simulink model "mrefrobotarm_modified_previous_y_previous_u_previous_ref"  (R2018b)
settings: Solver=FixedStepAuto  StartTime=0.0  StopTime=10  RelTol=1e-3  AbsTol=1e-6
undefined symbols (not defined in the file or in its folder): options, sfunxy2
libraries: neural x949, simulink x1
(part 10 of 31)

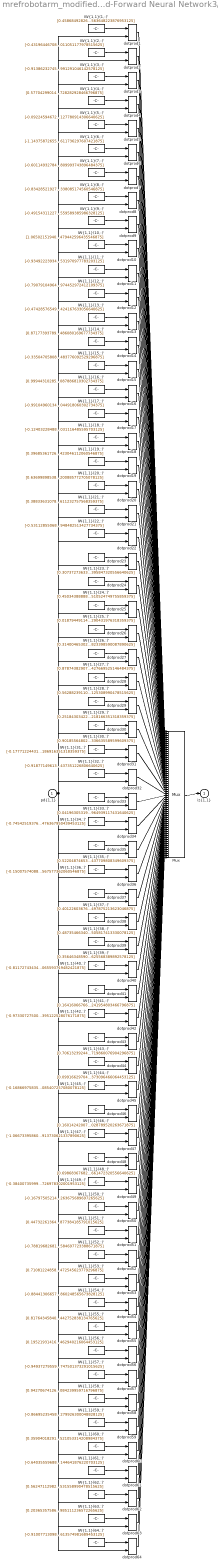
== system mrefrobotarm_modified_previous_y_previous_u_previous_ref/Feed-Forward Neural Network3/Layer 1/IW{1,1} ==
  "pd{1,1}" : Inport  PortDimensions=10
      mask Display: e = 0.06;c1 = [120 230 180]/255;c2 = ([120 230 180]+0)/(256+128);c3 = ([120 230 180]+128)/(256+128);patch([0 1 1 0],[0 0 1 1],c1);patch([0 1 1 1-e 1-e 0+e],[0 0 1 1-e 0+e 0+e],c2);patch([0 0 1 1-e 0+e 0+e],[0 1 1 1-e 1-e 0+e],c3);plot([0 1 1 0 0],[0 0 1 1 0]);
  "IW{1,1}(1,:)'" : Constant  Value=[0.45868492826623252778261985440622083842754364013671875;0.92289285731776471433107644770643673837184906005859375;-0.9045151079076070299578304911847226321697235107421875;0.6809770305948614765867432652157731354236602783203125;0.087608306906038213579535067765391431748867034912109375;-0.66859815839908964818505410221405327320098876953125;0.59153382468235282676261022061225958168506622314453125;0.66963699792932296350755905223195441067218780517578125;-0.464262938377100364828464762467774562537670135498046875;0.56319562975735781851227557126549072563648223876953125]
      mask Display: e = 0.06;c1 = [120 150 230]/255;c2 = ([120 150 230]+0)/383;c3 = ([120 150 230]+128)/383;patch([0 1 1 0],[0 0 1 1],c1);patch([0 1 1 1-e 1-e 0+e],[0 0 1 1-e 0+e 0+e],c2);patch([0 0 1 1-e 0+e 0+e],[0 1 1 1-e 1-e 0+e],c3);plot([0 1 1 0 0],[0 0 1 1 0]);disp('Weights');
  "IW{1,1}(10,:)'" : Constant  Value=[1.0650215194068157753548575783497653901576995849609375;0.923145532654704226160902180708944797515869140625;-0.28571602112830019049027896471670828759670257568359375;0.2206176877894590881989955732933594845235347747802734375;0.391759031266789181646714723683544434607028961181640625;0.4150000499566035561116450480767525732517242431640625;0.860171860662010789866371851530857384204864501953125;0.0858881248601063573833158670822740532457828521728515625;0.5686673804248325581056633382104337215423583984375;-0.8955203949568850685380994036677293479442596435546875]
      mask Display: e = 0.06;c1 = [120 150 230]/255;c2 = ([120 150 230]+0)/383;c3 = ([120 150 230]+128)/383;patch([0 1 1 0],[0 0 1 1],c1);patch([0 1 1 1-e 1-e 0+e],[0 0 1 1-e 0+e 0+e],c2);patch([0 0 1 1-e 0+e 0+e],[0 1 1 1-e 1-e 0+e],c3);plot([0 1 1 0 0],[0 0 1 1 0]);disp('Weights');
  "IW{1,1}(11,:)'" : Constant  Value=[-0.93492223934107243632496420104871504008769989013671875;0.356879505478416347852288481590221635997295379638671875;-0.042209624670428151638201796913563157431781291961669921875;0.6022490918690073247176997028873302042484283447265625;-1.3686982846566972948920692942920140922069549560546875;0.40979658750527558908061109832488000392913818359375;0.1714981863599602529557586194641771726310253143310546875;-0.75640045003631828368639844484278000891208648681640625;-0.12006348380912713891266463406282127834856510162353515625;0.632123796732191323144434136338531970977783203125]
      mask Display: e = 0.06;c1 = [120 150 230]/255;c2 = ([120 150 230]+0)/383;c3 = ([120 150 230]+128)/383;patch([0 1 1 0],[0 0 1 1],c1);patch([0 1 1 1-e 1-e 0+e],[0 0 1 1-e 0+e 0+e],c2);patch([0 0 1 1-e 0+e 0+e],[0 1 1 1-e 1-e 0+e],c3);plot([0 1 1 0 0],[0 0 1 1 0]);disp('Weights');
  "IW{1,1}(12,:)'" : Constant  Value=[-0.790791049648713606501360118272714316844940185546875;1.636635942456649228660126027534715831279754638671875;0.1645966634930366712108451565654831938445568084716796875;0.423800984374966327461464743464603088796138763427734375;-0.480947159258651557589558933614171110093593597412109375;-0.336459083953336790528965138946659862995147705078125;-0.29103815338116156841152815104578621685504913330078125;0.36537606798097732596630748957977630198001861572265625;0.5351649818216219767208485791343264281749725341796875;-0.360421095733105933955897626219666562974452972412109375]
      mask Display: e = 0.06;c1 = [120 150 230]/255;c2 = ([120 150 230]+0)/383;c3 = ([120 150 230]+128)/383;patch([0 1 1 0],[0 0 1 1],c1);patch([0 1 1 1-e 1-e 0+e],[0 0 1 1-e 0+e 0+e],c2);patch([0 0 1 1-e 0+e 0+e],[0 1 1 1-e 1-e 0+e],c3);plot([0 1 1 0 0],[0 0 1 1 0]);disp('Weights');
  "IW{1,1}(13,:)'" : Constant  Value=[-0.47428576549192869027393726355512626469135284423828125;0.481480766900708678779352567289606668055057525634765625;0.73462601397020887983302372958860360085964202880859375;-0.759579012370747985727348350337706506252288818359375;-2.289916762842977959735435433685779571533203125;-0.1033609967207107793729647937652771361172199249267578125;-1.0397695114935359139707315989653579890727996826171875;-0.11461751153739645203710750820391695015132427215576171875;0.607068239082933391870255945832468569278717041015625;0.627700190232618471242176383384503424167633056640625]
      mask Display: e = 0.06;c1 = [120 150 230]/255;c2 = ([120 150 230]+0)/383;c3 = ([120 150 230]+128)/383;patch([0 1 1 0],[0 0 1 1],c1);patch([0 1 1 1-e 1-e 0+e],[0 0 1 1-e 0+e 0+e],c2);patch([0 0 1 1-e 0+e 0+e],[0 1 1 1-e 1-e 0+e],c3);plot([0 1 1 0 0],[0 0 1 1 0]);disp('Weights');
  "IW{1,1}(14,:)'" : Constant  Value=[0.87177393789064960838430806688847951591014862060546875;-0.4062935623759871273108501554816029965877532958984375;-0.184561604501509435305450779196689836680889129638671875;-0.30955013114295903964290346266352571547031402587890625;-1.07748704376167214746828904026187956333160400390625;0.5280876054022181076419428791268728673458099365234375;-0.9211683717671104165702899990719743072986602783203125;0.4257168604823367008549439560738392174243927001953125;-0.9567072022642946205195357833872549235820770263671875;0.72989237124469974471452360376133583486080169677734375]
      mask Display: e = 0.06;c1 = [120 150 230]/255;c2 = ([120 150 230]+0)/383;c3 = ([120 150 230]+128)/383;patch([0 1 1 0],[0 0 1 1],c1);patch([0 1 1 1-e 1-e 0+e],[0 0 1 1-e 0+e 0+e],c2);patch([0 0 1 1-e 0+e 0+e],[0 1 1 1-e 1-e 0+e],c3);plot([0 1 1 0 0],[0 0 1 1 0]);disp('Weights');
  "IW{1,1}(15,:)'" : Constant  Value=[-0.335047058088355165228477972050313837826251983642578125;0.20537436519986662641912289473111741244792938232421875;-0.370389460774058376646422630074084736406803131103515625;-1.0764725130322230217672085927915759384632110595703125;0.9400904265613887478281185394735075533390045166015625;-0.90491999311588988685883805374032817780971527099609375;0.270630872633476904365323889578576199710369110107421875;0.7130288673092282092369487145333550870418548583984375;0.635657126622342527610953766270540654659271240234375;0.049580374452241053606638132578154909424483776092529296875]
      mask Display: e = 0.06;c1 = [120 150 230]/255;c2 = ([120 150 230]+0)/383;c3 = ([120 150 230]+128)/383;patch([0 1 1 0],[0 0 1 1],c1);patch([0 1 1 1-e 1-e 0+e],[0 0 1 1-e 0+e 0+e],c2);patch([0 0 1 1-e 0+e 0+e],[0 1 1 1-e 1-e 0+e],c3);plot([0 1 1 0 0],[0 0 1 1 0]);disp('Weights');
  "IW{1,1}(16,:)'" : Constant  Value=[0.9994431028540848860330925162998028099536895751953125;-0.07201816354893468552500479518130305223166942596435546875;0.9869266919961894313217953822459094226360321044921875;-0.037193845598922033179878354758329805918037891387939453125;0.0896492565684388897917500571566051803529262542724609375;0.030134033081079487914610837151485611684620380401611328125;0.57507766525746728536461205294472165405750274658203125;0.95965429457013395886377793431165628135204315185546875;-0.65200310057389998519283835776150226593017578125;0.7715891597542761104477904154919087886810302734375]
      mask Display: e = 0.06;c1 = [120 150 230]/255;c2 = ([120 150 230]+0)/383;c3 = ([120 150 230]+128)/383;patch([0 1 1 0],[0 0 1 1],c1);patch([0 1 1 1-e 1-e 0+e],[0 0 1 1-e 0+e 0+e],c2);patch([0 0 1 1-e 0+e 0+e],[0 1 1 1-e 1-e 0+e],c3);plot([0 1 1 0 0],[0 0 1 1 0]);disp('Weights');
  "IW{1,1}(17,:)'" : Constant  Value=[-0.991049601348017450419547458295710384845733642578125;0.1767823626110802404109989538483205251395702362060546875;-0.77042637580729300683657356785261072218418121337890625;1.0369587591067332965621972107328474521636962890625;-0.8204067837491482162448619419592432677745819091796875;-0.8007430151625019032479713132488541305065155029296875;0.09562009879907318321556886075995862483978271484375;-0.55794220575710007370417997663025744259357452392578125;0.663058379158372179773550669779069721698760986328125;0.12039199732993309532869119493625476025044918060302734375]
      mask Display: e = 0.06;c1 = [120 150 230]/255;c2 = ([120 150 230]+0)/383;c3 = ([120 150 230]+128)/383;patch([0 1 1 0],[0 0 1 1],c1);patch([0 1 1 1-e 1-e 0+e],[0 0 1 1-e 0+e 0+e],c2);patch([0 0 1 1-e 0+e 0+e],[0 1 1 1-e 1-e 0+e],c3);plot([0 1 1 0 0],[0 0 1 1 0]);disp('Weights');
  "IW{1,1}(18,:)'" : Constant  Value=[-0.12403228488311750232764296697496320120990276336669921875;-0.856750459537330311121650083805434405803680419921875;0.192918443102331804706039974917075596749782562255859375;1.03664335999274204169751101289875805377960205078125;-0.246904966516503676654537002832512371242046356201171875;-1.04666463077165872164187021553516387939453125;-0.033336987951685347064678666129111661575734615325927734375;0.855943230966101253898159484378993511199951171875;0.249998464760956162766802890473627485334873199462890625;0.71561037633987834016835449801874347031116485595703125]
      mask Display: e = 0.06;c1 = [120 150 230]/255;c2 = ([120 150 230]+0)/383;c3 = ([120 150 230]+128)/383;patch([0 1 1 0],[0 0 1 1],c1);patch([0 1 1 1-e 1-e 0+e],[0 0 1 1-e 0+e 0+e],c2);patch([0 0 1 1-e 0+e 0+e],[0 1 1 1-e 1-e 0+e],c3);plot([0 1 1 0 0],[0 0 1 1 0]);disp('Weights');
  "IW{1,1}(19,:)'" : Constant  Value=[0.39685361726252110781132387273828499019145965576171875;-0.7385100253306242645834345239563845098018646240234375;-0.032023900811615581274427455582554102875292301177978515625;-1.0360471954462855403988896796363405883312225341796875;0.024414108875345917615273805267861462198197841644287109375;-0.54557027817496128729857218786492012441158294677734375;-0.825321885041145009154206491075456142425537109375;-0.4206523039094769433887677223538048565387725830078125;-0.9226889362967900520828834487474523484706878662109375;0.5855123554608023805911898307385854423046112060546875]
      mask Display: e = 0.06;c1 = [120 150 230]/255;c2 = ([120 150 230]+0)/383;c3 = ([120 150 230]+128)/383;patch([0 1 1 0],[0 0 1 1],c1);patch([0 1 1 1-e 1-e 0+e],[0 0 1 1-e 0+e 0+e],c2);patch([0 0 1 1-e 0+e 0+e],[0 1 1 1-e 1-e 0+e],c3);plot([0 1 1 0 0],[0 0 1 1 0]);disp('Weights');
  "IW{1,1}(2,:)'" : Constant  Value=[-0.4319644670862052837634337265626527369022369384765625;1.131663563801270644404439735808409750461578369140625;-0.3687061577706416404254241570015437901020050048828125;-0.366144655751171221869100236290250904858112335205078125;-1.1602768057870693763078406846034340560436248779296875;0.1935191644854985237866884517643484286963939666748046875;-1.1688198788845378661704899059259332716464996337890625;0.59642228088652526896140670942259021103382110595703125;-0.213316011820075479565872456078068353235721588134765625;-0.60843334155029238363709964687586762011051177978515625]
      mask Display: e = 0.06;c1 = [120 150 230]/255;c2 = ([120 150 230]+0)/383;c3 = ([120 150 230]+128)/383;patch([0 1 1 0],[0 0 1 1],c1);patch([0 1 1 1-e 1-e 0+e],[0 0 1 1-e 0+e 0+e],c2);patch([0 0 1 1-e 0+e 0+e],[0 1 1 1-e 1-e 0+e],c3);plot([0 1 1 0 0],[0 0 1 1 0]);disp('Weights');
  "IW{1,1}(20,:)'" : Constant  Value=[0.63699898538872490316720131886540912091732025146484375;1.22411360040730965437205668422393500804901123046875;-0.2390034119129008927107093995800823904573917388916015625;-0.4946309213569535234711338489432819187641143798828125;-0.310348111937733095455627108094631694257259368896484375;0.64481659009713354624437897655298002064228057861328125;-0.406894473883987861650979311889386735856533050537109375;-0.75915863551750917270766194633324630558490753173828125;-0.9316675248445800416874362781527452170848846435546875;0.4791981902970114948203672611271031200885772705078125]
      mask Display: e = 0.06;c1 = [120 150 230]/255;c2 = ([120 150 230]+0)/383;c3 = ([120 150 230]+128)/383;patch([0 1 1 0],[0 0 1 1],c1);patch([0 1 1 1-e 1-e 0+e],[0 0 1 1-e 0+e 0+e],c2);patch([0 0 1 1-e 0+e 0+e],[0 1 1 1-e 1-e 0+e],c3);plot([0 1 1 0 0],[0 0 1 1 0]);disp('Weights');
  "IW{1,1}(21,:)'" : Constant  Value=[0.38833631078315045126458926461054943501949310302734375;-0.477922123057430703330084043045644648373126983642578125;-0.480202975146608534995351647012284956872463226318359375;-0.55323452941971229535056409076787531375885009765625;0.9656831493714037595310628603328950703144073486328125;-0.77207012724652568369521077329409308731555938720703125;0.819346846772037284978296156623400747776031494140625;1.237663352466707333832118820282630622386932373046875;-0.33134863320223384430818214241298846900463104248046875;-0.3405186420123695878459102459601126611232757568359375]
      mask Display: e = 0.06;c1 = [120 150 230]/255;c2 = ([120 150 230]+0)/383;c3 = ([120 150 230]+128)/383;patch([0 1 1 0],[0 0 1 1],c1);patch([0 1 1 1-e 1-e 0+e],[0 0 1 1-e 0+e 0+e],c2);patch([0 0 1 1-e 0+e 0+e],[0 1 1 1-e 1-e 0+e],c3);plot([0 1 1 0 0],[0 0 1 1 0]);disp('Weights');
  "IW{1,1}(22,:)'" : Constant  Value=[-0.53112855068060838004129209366510622203350067138671875;0.41770532386455538897962469491176307201385498046875;0.877645280928558424449192898464389145374298095703125;0.71215987560110016740821947678341530263423919677734375;-0.762781721122099298781904508359730243682861328125;0.5052308643133749388454134532366879284381866455078125;0.70107445065553763985377599965431727468967437744140625;0.9375496189941594504801969378604553639888763427734375;0.1867677108731029267385537195877986960113048553466796875;0.65377202488005303759877051561488769948482513427734375]
      mask Display: e = 0.06;c1 = [120 150 230]/255;c2 = ([120 150 230]+0)/383;c3 = ([120 150 230]+128)/383;patch([0 1 1 0],[0 0 1 1],c1);patch([0 1 1 1-e 1-e 0+e],[0 0 1 1-e 0+e 0+e],c2);patch([0 0 1 1-e 0+e 0+e],[0 1 1 1-e 1-e 0+e],c3);plot([0 1 1 0 0],[0 0 1 1 0]);disp('Weights');
  "IW{1,1}(23,:)'" : Constant  Value=[0.307372736331202711657084591934108175337314605712890625;-0.05892926126433717382013810492935590445995330810546875;-0.8454741438367745498538852189085446298122406005859375;-0.90214871964219345290558749184128828346729278564453125;0.52882827674761923031354626800748519599437713623046875;-0.91735938960778806716689359745942056179046630859375;0.439037397626755587776159472923609428107738494873046875;-0.8401705313617597870035069718142040073871612548828125;-0.68098266724226419466248216849635355174541473388671875;-0.6560593294393444185885755359777249395847320556640625]
      mask Display: e = 0.06;c1 = [120 150 230]/255;c2 = ([120 150 230]+0)/383;c3 = ([120 150 230]+128)/383;patch([0 1 1 0],[0 0 1 1],c1);patch([0 1 1 1-e 1-e 0+e],[0 0 1 1-e 0+e 0+e],c2);patch([0 0 1 1-e 0+e 0+e],[0 1 1 1-e 1-e 0+e],c3);plot([0 1 1 0 0],[0 0 1 1 0]);disp('Weights');
  "IW{1,1}(24,:)'" : Constant  Value=[0.4503438888826376551577368445578031241893768310546875;0.7786736499867739080826822828385047614574432373046875;-0.1252306288409761325652880259440280497074127197265625;-0.377179788931731818646397869088104926049709320068359375;0.56682512736796419883233966174884699285030364990234375;0.7596722035946166240449883844121359288692474365234375;-1.1299355991591040204724549766979180276393890380859375;-0.30400712082542213909874817545642144978046417236328125;1.0664004939714619712987087041256017982959747314453125;-0.20735732554729435772600254495046101510524749755859375]
      mask Display: e = 0.06;c1 = [120 150 230]/255;c2 = ([120 150 230]+0)/383;c3 = ([120 150 230]+128)/383;patch([0 1 1 0],[0 0 1 1],c1);patch([0 1 1 1-e 1-e 0+e],[0 0 1 1-e 0+e 0+e],c2);patch([0 0 1 1-e 0+e 0+e],[0 1 1 1-e 1-e 0+e],c3);plot([0 1 1 0 0],[0 0 1 1 0]);disp('Weights');
  "IW{1,1}(25,:)'" : Constant  Value=[0.0187944911497716395099022435033475630916655063629150390625;-0.29171160022622633078981380094774067401885986328125;-0.6290327137339668528426273041986860334873199462890625;-0.60111063940849718267855905651231296360492706298828125;-0.84503479054379526669293909435509704053401947021484375;1.00065376837120112440970842726528644561767578125;-1.0220616759307910026421950533404015004634857177734375;0.23813155884114645122195952353649772703647613525390625;0.58258232582170721425285364603041671216487884521484375;-0.2077397536722867810166093249790719710290431976318359375]
      mask Display: e = 0.06;c1 = [120 150 230]/255;c2 = ([120 150 230]+0)/383;c3 = ([120 150 230]+128)/383;patch([0 1 1 0],[0 0 1 1],c1);patch([0 1 1 1-e 1-e 0+e],[0 0 1 1-e 0+e 0+e],c2);patch([0 0 1 1-e 0+e 0+e],[0 1 1 1-e 1-e 0+e],c3);plot([0 1 1 0 0],[0 0 1 1 0]);disp('Weights');
  "IW{1,1}(26,:)'" : Constant  Value=[0.314004653024913926717687218115315772593021392822265625;0.28496225052615298256597498038900084793567657470703125;-0.020555819018938083220238155490733333863317966461181640625;-0.768406212368593966033358810818754136562347412109375;-0.702615478109754665325681344256736338138580322265625;-1.189394172537658445065744672319851815700531005859375;-0.90344082742903542015966422695782966911792755126953125;-0.282389771335746553315715345888747833669185638427734375;0.06348411509587427448142449293300160206854343414306640625;0.3946538105354913117395199151360429823398590087890625]
      mask Display: e = 0.06;c1 = [120 150 230]/255;c2 = ([120 150 230]+0)/383;c3 = ([120 150 230]+128)/383;patch([0 1 1 0],[0 0 1 1],c1);patch([0 1 1 1-e 1-e 0+e],[0 0 1 1-e 0+e 0+e],c2);patch([0 0 1 1-e 0+e 0+e],[0 1 1 1-e 1-e 0+e],c3);plot([0 1 1 0 0],[0 0 1 1 0]);disp('Weights');
  "IW{1,1}(27,:)'" : Constant  Value=[0.87874382907473036485868078671046532690525054931640625;0.60810217822310008717323626115103252232074737548828125;-0.292770568818674081779107609690981917083263397216796875;-1.0529162479607714342222379855229519307613372802734375;-0.65486630135451984191519159139716066420078277587890625;-0.797220628919749874086164709297008812427520751953125;0.1839437904078597696422292528950492851436138153076171875;-0.1829250381180290430105372934121987782418727874755859375;-0.333508322957326963642543660171213559806346893310546875;0.73330763357021933046553385793231427669525146484375]
      mask Display: e = 0.06;c1 = [120 150 230]/255;c2 = ([120 150 230]+0)/383;c3 = ([120 150 230]+128)/383;patch([0 1 1 0],[0 0 1 1],c1);patch([0 1 1 1-e 1-e 0+e],[0 0 1 1-e 0+e 0+e],c2);patch([0 0 1 1-e 0+e 0+e],[0 1 1 1-e 1-e 0+e],c3);plot([0 1 1 0 0],[0 0 1 1 0]);disp('Weights');
  "IW{1,1}(28,:)'" : Constant  Value=[0.56288239110132021192356432948145084083080291748046875;-0.9167817868636156664052805354003794491291046142578125;-0.37108127426537418358520881156437098979949951171875;-0.94968441008708370798530040701734833419322967529296875;-0.828961314456096776126514669158495962619781494140625;-0.34260164506463797184920849758782424032688140869140625;0.56198258845486204204888736057910136878490447998046875;0.463369775931001648405782589179580099880695343017578125;0.89346008209063698668472852659760974347591400146484375;-0.37152484249957906659034279073239304125308990478515625]
      mask Display: e = 0.06;c1 = [120 150 230]/255;c2 = ([120 150 230]+0)/383;c3 = ([120 150 230]+128)/383;patch([0 1 1 0],[0 0 1 1],c1);patch([0 1 1 1-e 1-e 0+e],[0 0 1 1-e 0+e 0+e],c2);patch([0 0 1 1-e 0+e 0+e],[0 1 1 1-e 1-e 0+e],c3);plot([0 1 1 0 0],[0 0 1 1 0]);disp('Weights');
  "IW{1,1}(29,:)'" : Constant  Value=[0.251843034229094986375940834477660246193408966064453125;-0.307514231193741272019082089173025451600551605224609375;1.017125500204711929796985714347101747989654541015625;0.460524441656800342936861625275923870503902435302734375;0.79131721944803856683137155414442531764507293701171875;0.57246841923376201588524736507679335772991180419921875;0.7128468337145701383406048989854753017425537109375;-0.63645636262505400626565688071423210203647613525390625;-0.74370154532832533078590131481178104877471923828125;0.32549381312921976672214441350661218166351318359375]
      mask Display: e = 0.06;c1 = [120 150 230]/255;c2 = ([120 150 230]+0)/383;c3 = ([120 150 230]+128)/383;patch([0 1 1 0],[0 0 1 1],c1);patch([0 1 1 1-e 1-e 0+e],[0 0 1 1-e 0+e 0+e],c2);patch([0 0 1 1-e 0+e 0+e],[0 1 1 1-e 1-e 0+e],c3);plot([0 1 1 0 0],[0 0 1 1 0]);disp('Weights');
  "IW{1,1}(3,:)'" : Constant  Value=[-0.91386232745777451480506670122849754989147186279296875;-0.45074517661076374253070753184147179126739501953125;0.7779681185418085842542268437682650983333587646484375;0.301880156597266358087239268570556305348873138427734375;-0.36510036078684515725711889899685047566890716552734375;0.435149932138041872775602314504794776439666748046875;0.744516076638678470089871552772819995880126953125;0.79936263013440156388611512738862074911594390869140625;-0.9761044371817184650552690072800032794475555419921875;0.09260100631979346907929340204645995981991291046142578125]
      mask Display: e = 0.06;c1 = [120 150 230]/255;c2 = ([120 150 230]+0)/383;c3 = ([120 150 230]+128)/383;patch([0 1 1 0],[0 0 1 1],c1);patch([0 1 1 1-e 1-e 0+e],[0 0 1 1-e 0+e 0+e],c2);patch([0 0 1 1-e 0+e 0+e],[0 1 1 1-e 1-e 0+e],c3);plot([0 1 1 0 0],[0 0 1 1 0]);disp('Weights');
  "IW{1,1}(30,:)'" : Constant  Value=[0.9018556480275676801028339468757621943950653076171875;-0.78729557282458861866558663678006269037723541259765625;-0.019885436964666249048949708821965032257139682769775390625;0.052447295981474760517837552242781384848058223724365234375;-0.889009231846008329824826432741247117519378662109375;-0.9610547041058754569320399241405539214611053466796875;-0.182018297743394119603266290141618810594081878662109375;0.72526023146258944418462988323881290853023529052734375;0.64039996155931699917118748999200761318206787109375;0.1507741773735079282570126224527484737336635589599609375]
      mask Display: e = 0.06;c1 = [120 150 230]/255;c2 = ([120 150 230]+0)/383;c3 = ([120 150 230]+128)/383;patch([0 1 1 0],[0 0 1 1],c1);patch([0 1 1 1-e 1-e 0+e],[0 0 1 1-e 0+e 0+e],c2);patch([0 0 1 1-e 0+e 0+e],[0 1 1 1-e 1-e 0+e],c3);plot([0 1 1 0 0],[0 0 1 1 0]);disp('Weights');
  "IW{1,1}(31,:)'" : Constant  Value=[-0.177712244314512435305886128844576887786388397216796875;-1.2044180642528250491096741825458593666553497314453125;0.476297722669175194187829447400872595608234405517578125;1.027514245695015038251085570664145052433013916015625;0.301166659778433432048672102609998546540737152099609375;-0.75506722651343294305803510724217630922794342041015625;0.07699562646007508670553676211056881584227085113525390625;0.384843310822156225992074496389250271022319793701171875;0.285367648969371945355533171095885336399078369140625;-1.126896382412153396757048540166579186916351318359375]
      mask Display: e = 0.06;c1 = [120 150 230]/255;c2 = ([120 150 230]+0)/383;c3 = ([120 150 230]+128)/383;patch([0 1 1 0],[0 0 1 1],c1);patch([0 1 1 1-e 1-e 0+e],[0 0 1 1-e 0+e 0+e],c2);patch([0 0 1 1-e 0+e 0+e],[0 1 1 1-e 1-e 0+e],c3);plot([0 1 1 0 0],[0 0 1 1 0]);disp('Weights');
  "IW{1,1}(32,:)'" : Constant  Value=[-0.91877149613463160449100541882216930389404296875;-0.7041488799692736666457903993432410061359405517578125;-0.6902299079520906044393768752343021333217620849609375;0.181024345450790935529994385433383285999298095703125;0.8149545053124309657022195096942596137523651123046875;-0.188996880097075659055150254062027670443058013916015625;0.5324856393693753187079664712655358016490936279296875;0.66680255622811468452226790759596042335033416748046875;-0.325096445121553834223249168644542805850505828857421875;0.72295756338197580959104016073979437351226806640625]
      mask Display: e = 0.06;c1 = [120 150 230]/255;c2 = ([120 150 230]+0)/383;c3 = ([120 150 230]+128)/383;patch([0 1 1 0],[0 0 1 1],c1);patch([0 1 1 1-e 1-e 0+e],[0 0 1 1-e 0+e 0+e],c2);patch([0 0 1 1-e 0+e 0+e],[0 1 1 1-e 1-e 0+e],c3);plot([0 1 1 0 0],[0 0 1 1 0]);disp('Weights');
  "IW{1,1}(33,:)'" : Constant  Value=[0.04196305319293618107945320616636308841407299041748046875;0.76655853000515727924124576020403765141963958740234375;0.80603316035365557556957583074108697474002838134765625;-0.370158384866360989917666302062571048736572265625;-0.6648584293383577037417353494674898684024810791015625;-1.088403289602522416856800191453658044338226318359375;-0.5881887256931204177590188919566571712493896484375;0.463144574540498898951312867211527191102504730224609375;-0.7447264394515855645551027919282205402851104736328125;-0.63389040345143998766985760084935463964939117431640625]
      mask Display: e = 0.06;c1 = [120 150 230]/255;c2 = ([120 150 230]+0)/383;c3 = ([120 150 230]+128)/383;patch([0 1 1 0],[0 0 1 1],c1);patch([0 1 1 1-e 1-e 0+e],[0 0 1 1-e 0+e 0+e],c2);patch([0 0 1 1-e 0+e 0+e],[0 1 1 1-e 1-e 0+e],c3);plot([0 1 1 0 0],[0 0 1 1 0]);disp('Weights');
  "IW{1,1}(34,:)'" : Constant  Value=[-0.745425193763594950979722852935083210468292236328125;0.8437511723446655675928695927723310887813568115234375;-0.35519126498091413424162965384311974048614501953125;1.145983154683168692145045497454702854156494140625;-0.8181579621718093608961908103083260357379913330078125;0.34044035693652052732005586221930570900440216064453125;0.0200030161024008119874384448166892980225384235382080078125;0.56514643394315722257914558213087730109691619873046875;-0.639894538440779481192066668882034718990325927734375;0.62916251619793872595920447565731592476367950439453125]
      mask Display: e = 0.06;c1 = [120 150 230]/255;c2 = ([120 150 230]+0)/383;c3 = ([120 150 230]+128)/383;patch([0 1 1 0],[0 0 1 1],c1);patch([0 1 1 1-e 1-e 0+e],[0 0 1 1-e 0+e 0+e],c2);patch([0 0 1 1-e 0+e 0+e],[0 1 1 1-e 1-e 0+e],c3);plot([0 1 1 0 0],[0 0 1 1 0]);disp('Weights');
  "IW{1,1}(35,:)'" : Constant  Value=[0.5220487465308909502681444791960529983043670654296875;-0.38328664517104515940815190333523787558078765869140625;0.1705678755793129663942409024457447230815887451171875;-0.5505032642886000804338664238457567989826202392578125;0.91195652457662113032910156107391230762004852294921875;0.549813390225727172122560659772716462612152099609375;0.56085932523472081800974819998373277485370635986328125;-0.73311912984947580351757778771570883691310882568359375;-0.62407319091514212860971611007698811590671539306640625;1.043032154999939731254698926932178437709808349609375]
      mask Display: e = 0.06;c1 = [120 150 230]/255;c2 = ([120 150 230]+0)/383;c3 = ([120 150 230]+128)/383;patch([0 1 1 0],[0 0 1 1],c1);patch([0 1 1 1-e 1-e 0+e],[0 0 1 1-e 0+e 0+e],c2);patch([0 0 1 1-e 0+e 0+e],[0 1 1 1-e 1-e 0+e],c3);plot([0 1 1 0 0],[0 0 1 1 0]);disp('Weights');
  "IW{1,1}(36,:)'" : Constant  Value=[-0.1500757408864716868635014179744757711887359619140625;-0.923805194473154234202638690476305782794952392578125;-0.392113893842136518319563265322358347475528717041015625;0.8983622595558229395606986145139671862125396728515625;-0.73945226212211079275249403508496470749378204345703125;0.73171210756552962362064818080398254096508026123046875;-0.5093700522200486080492964902077801525592803955078125;0.234384945730751137471514766730251722037792205810546875;0.98605141966327536362513228596071712672710418701171875;-0.390524721104801908477810457043233327567577362060546875]
      mask Display: e = 0.06;c1 = [120 150 230]/255;c2 = ([120 150 230]+0)/383;c3 = ([120 150 230]+128)/383;patch([0 1 1 0],[0 0 1 1],c1);patch([0 1 1 1-e 1-e 0+e],[0 0 1 1-e 0+e 0+e],c2);patch([0 0 1 1-e 0+e 0+e],[0 1 1 1-e 1-e 0+e],c3);plot([0 1 1 0 0],[0 0 1 1 0]);disp('Weights');
  "IW{1,1}(37,:)'" : Constant  Value=[0.40122603676745061118680268918978981673717498779296875;0.9489721667510442326687325476086698472499847412109375;0.9650136349198590313136492113699205219745635986328125;-0.461708720525743576690302916176733560860157012939453125;0.462280823831634546383639872146886773407459259033203125;-0.302021292443089617307805383461527526378631591796875;-1.121888991919543610009668554994277656078338623046875;0.6085838231360647387901963156764395534992218017578125;0.09693985105834827809001552623158204369246959686279296875;0.5949016996355733777335217382642440497875213623046875]
      mask Display: e = 0.06;c1 = [120 150 230]/255;c2 = ([120 150 230]+0)/383;c3 = ([120 150 230]+128)/383;patch([0 1 1 0],[0 0 1 1],c1);patch([0 1 1 1-e 1-e 0+e],[0 0 1 1-e 0+e 0+e],c2);patch([0 0 1 1-e 0+e 0+e],[0 1 1 1-e 1-e 0+e],c3);plot([0 1 1 0 0],[0 0 1 1 0]);disp('Weights');
  "IW{1,1}(38,:)'" : Constant  Value=[0.48735466340841171462017200610716827213764190673828125;0.1660571009135219655572512920116423629224300384521484375;0.98444903279443429777728624685551039874553680419921875;-0.58142103790658816730996250043972395360469818115234375;-0.81514060009158650910165988534572534263134002685546875;0.8406389862650691657819379543070681393146514892578125;0.09088775929998775537921318345979670993983745574951171875;0.711748564614161249863855118746869266033172607421875;-0.258756314964575295789472875185310840606689453125;-0.95815111970322697221291718960856087505817413330078125]
      mask Display: e = 0.06;c1 = [120 150 230]/255;c2 = ([120 150 230]+0)/383;c3 = ([120 150 230]+128)/383;patch([0 1 1 0],[0 0 1 1],c1);patch([0 1 1 1-e 1-e 0+e],[0 0 1 1-e 0+e 0+e],c2);patch([0 0 1 1-e 0+e 0+e],[0 1 1 1-e 1-e 0+e],c3);plot([0 1 1 0 0],[0 0 1 1 0]);disp('Weights');
  "IW{1,1}(39,:)'" : Constant  Value=[0.35646348590771481656958030725945718586444854736328125;-0.8942120032138476393157588972826488316059112548828125;0.499219065371001857744914786962908692657947540283203125;0.428384098335756247077910074949613772332668304443359375;-1.02259216879095315988479342195205390453338623046875;-0.8539655339702594272210944836842827498912811279296875;0.259630100426019694292989470341126434504985809326171875;-0.72381758717223110277672049051034264266490936279296875;0.1828645386369745218235749462110106833279132843017578125;-0.97010093673340680453520690207369625568389892578125]
      mask Display: e = 0.06;c1 = [120 150 230]/255;c2 = ([120 150 230]+0)/383;c3 = ([120 150 230]+128)/383;patch([0 1 1 0],[0 0 1 1],c1);patch([0 1 1 1-e 1-e 0+e],[0 0 1 1-e 0+e 0+e],c2);patch([0 0 1 1-e 0+e 0+e],[0 1 1 1-e 1-e 0+e],c3);plot([0 1 1 0 0],[0 0 1 1 0]);disp('Weights');
  "IW{1,1}(4,:)'" : Constant  Value=[0.57704299014256321687099671180476434528827667236328125;-0.3297771120958981061477288676542229950428009033203125;0.6499294520401475150350734111270867288112640380859375;0.5681734445177462067277929236297495663166046142578125;1.1424874290442026403269437651033513247966766357421875;0.32833120954897643262171413880423642694950103759765625;-0.74775060928833336770793493997189216315746307373046875;0.515259663239628906694633769802749156951904296875;0.8974102410702686771770686391391791403293609619140625;-0.496963084017053080554404687063652090728282928466796875]
      mask Display: e = 0.06;c1 = [120 150 230]/255;c2 = ([120 150 230]+0)/383;c3 = ([120 150 230]+128)/383;patch([0 1 1 0],[0 0 1 1],c1);patch([0 1 1 1-e 1-e 0+e],[0 0 1 1-e 0+e 0+e],c2);patch([0 0 1 1-e 0+e 0+e],[0 1 1 1-e 1-e 0+e],c3);plot([0 1 1 0 0],[0 0 1 1 0]);disp('Weights');
  "IW{1,1}(40,:)'" : Constant  Value=[-0.8117274343416946980056536631309427320957183837890625;-1.065920559880181084366768118343316018581390380859375;0.51720231546692574386980822964687831699848175048828125;-0.434361952170224940861231743838288821280002593994140625;0.0190341195698830838167747714351207832805812358856201171875;0.367593061946847488030698514194227755069732666015625;-0.7189283397463122060599971518968231976032257080078125;-0.107753624986951901387755015093716792762279510498046875;1.0883766562623258256081726358388550579547882080078125;0.447296112987982830144773060965235345065593719482421875]
      mask Display: e = 0.06;c1 = [120 150 230]/255;c2 = ([120 150 230]+0)/383;c3 = ([120 150 230]+128)/383;patch([0 1 1 0],[0 0 1 1],c1);patch([0 1 1 1-e 1-e 0+e],[0 0 1 1-e 0+e 0+e],c2);patch([0 0 1 1-e 0+e 0+e],[0 1 1 1-e 1-e 0+e],c3);plot([0 1 1 0 0],[0 0 1 1 0]);disp('Weights');
  "IW{1,1}(41,:)'" : Constant  Value=[0.164160667665698090100789841017103753983974456787109375;0.95738171703772845244628797445329837501049041748046875;0.7062699381101247286807165437494404613971710205078125;0.399933604794525610071076471285778097808361053466796875;0.7171371306546976409634908122825436294078826904296875;-1.1202839080823354667160174358286894857883453369140625;-0.1853772287894561443533092415236751548945903778076171875;-0.74462254835949914788528758435859344899654388427734375;-0.50416859995003437955318759122746996581554412841796875;-0.420484155532803771659899894075351767241954803466796875]
      mask Display: e = 0.06;c1 = [120 150 230]/255;c2 = ([120 150 230]+0)/383;c3 = ([120 150 230]+128)/383;patch([0 1 1 0],[0 0 1 1],c1);patch([0 1 1 1-e 1-e 0+e],[0 0 1 1-e 0+e 0+e],c2);patch([0 0 1 1-e 0+e 0+e],[0 1 1 1-e 1-e 0+e],c3);plot([0 1 1 0 0],[0 0 1 1 0]);disp('Weights');
  "IW{1,1}(42,:)'" : Constant  Value=[-0.97330727500253766404370026066317223012447357177734375;-0.6376090744330138448958678054623305797576904296875;0.56613088501629127424763510134653188288211822509765625;0.66429044491389854787399826818727888166904449462890625;0.63823090480270783242389143197215162217617034912109375;0.89940392939894631130215429948293603956699371337890625;-0.426425485051496966359962925707804970443248748779296875;0.77548507787086062847947687259875237941741943359375;-0.2005345463581615639281352514444733969867229461669921875;0.76065296756111322462601265215198509395122528076171875]
      mask Display: e = 0.06;c1 = [120 150 230]/255;c2 = ([120 150 230]+0)/383;c3 = ([120 150 230]+128)/383;patch([0 1 1 0],[0 0 1 1],c1);patch([0 1 1 1-e 1-e 0+e],[0 0 1 1-e 0+e 0+e],c2);patch([0 0 1 1-e 0+e 0+e],[0 1 1 1-e 1-e 0+e],c3);plot([0 1 1 0 0],[0 0 1 1 0]);disp('Weights');
  "IW{1,1}(43,:)'" : Constant  Value=[0.70613239244119008208855348129873163998126983642578125;-0.0032671817422963238784772155298696816316805779933929443359375;0.367882464476378123752198234797106124460697174072265625;0.53716568114694995816904565799632109701633453369140625;-0.60385405900132227419163655213196761906147003173828125;0.56356107810884370490356332084047608077526092529296875;-1.2335498781115941113739609136246144771575927734375;-0.55756872644362676094687003569561056792736053466796875;0.68280368798035329103157664576428942382335662841796875;0.3513308387828206758030091805267147719860076904296875]
      mask Display: e = 0.06;c1 = [120 150 230]/255;c2 = ([120 150 230]+0)/383;c3 = ([120 150 230]+128)/383;patch([0 1 1 0],[0 0 1 1],c1);patch([0 1 1 1-e 1-e 0+e],[0 0 1 1-e 0+e 0+e],c2);patch([0 0 1 1-e 0+e 0+e],[0 1 1 1-e 1-e 0+e],c3);plot([0 1 1 0 0],[0 0 1 1 0]);disp('Weights');
  "IW{1,1}(44,:)'" : Constant  Value=[0.0991662970499278817460009349815663881599903106689453125;-0.23734506227607410355773254195810295641422271728515625;0.62818548146802388743026313022710382938385009765625;-0.9129688653862937375293995501124300062656402587890625;-0.2172478617775137343937075229405309073626995086669921875;-0.01335464061911364151702397151666446006856858730316162109375;1.137547187144944960124348654062487185001373291015625;1.0483013182981137934035587022663094103336334228515625;-0.31625374105714298966773867505253292620182037353515625;-0.80021297976558447562211995318648405373096466064453125]
      mask Display: e = 0.06;c1 = [120 150 230]/255;c2 = ([120 150 230]+0)/383;c3 = ([120 150 230]+128)/383;patch([0 1 1 0],[0 0 1 1],c1);patch([0 1 1 1-e 1-e 0+e],[0 0 1 1-e 0+e 0+e],c2);patch([0 0 1 1-e 0+e 0+e],[0 1 1 1-e 1-e 0+e],c3);plot([0 1 1 0 0],[0 0 1 1 0]);disp('Weights');
  "IW{1,1}(45,:)'" : Constant  Value=[-0.1686697583546842571511348296553478576242923736572265625;0.525569051946446652578970315516926348209381103515625;-0.7477028093603312886017420169082470238208770751953125;0.748042650913563367254255354055203497409820556640625;0.9218607481481113641308411388308741152286529541015625;-0.395022844379094129063645368660218082368373870849609375;-0.92733777555402951975338510237634181976318359375;0.0132672175676092247986748162702497211284935474395751953125;0.8182811397371494432917415906558744609355926513671875;-0.71927847455369964269067395434831269085407257080078125]
      mask Display: e = 0.06;c1 = [120 150 230]/255;c2 = ([120 150 230]+0)/383;c3 = ([120 150 230]+128)/383;patch([0 1 1 0],[0 0 1 1],c1);patch([0 1 1 1-e 1-e 0+e],[0 0 1 1-e 0+e 0+e],c2);patch([0 0 1 1-e 0+e 0+e],[0 1 1 1-e 1-e 0+e],c3);plot([0 1 1 0 0],[0 0 1 1 0]);disp('Weights');
  "IW{1,1}(46,:)'" : Constant  Value=[0.1601424200775466155644011223557754419744014739990234375;-0.47571559161783427693848125272779725492000579833984375;0.390102210125831183606948115993873216211795806884765625;-0.545689954050754710834780780714936554431915283203125;-0.1706928204696639694848414592343033291399478912353515625;1.021403706467001626378987566567957401275634765625;-0.820522700882862832116870777099393308162689208984375;-1.1603263281579307975022175014601089060306549072265625;-0.1083543434952064787868408757276483811438083648681640625;-0.9782316390368464009696936045656912028789520263671875]
      mask Display: e = 0.06;c1 = [120 150 230]/255;c2 = ([120 150 230]+0)/383;c3 = ([120 150 230]+128)/383;patch([0 1 1 0],[0 0 1 1],c1);patch([0 1 1 1-e 1-e 0+e],[0 0 1 1-e 0+e 0+e],c2);patch([0 0 1 1-e 0+e 0+e],[0 1 1 1-e 1-e 0+e],c3);plot([0 1 1 0 0],[0 0 1 1 0]);disp('Weights');
  "IW{1,1}(47,:)'" : Constant  Value=[-1.0667339586099202630720128581742756068706512451171875;0.78778700900907894233426986829726956784725189208984375;0.42322582107684547647608042097999714314937591552734375;0.486047035425058504554129967800690792500972747802734375;-0.056824286572496336689130913555345614440739154815673828125;0.84373266382901757065582160066696815192699432373046875;-1.0525997952128711698804863772238604724407196044921875;0.50240107206545936424646470186416991055011749267578125;-0.263094040207939083853005968194338493049144744873046875;0.90872746411031679603098609732114709913730621337890625]
      mask Display: e = 0.06;c1 = [120 150 230]/255;c2 = ([120 150 230]+0)/383;c3 = ([120 150 230]+128)/383;patch([0 1 1 0],[0 0 1 1],c1);patch([0 1 1 1-e 1-e 0+e],[0 0 1 1-e 0+e 0+e],c2);patch([0 0 1 1-e 0+e 0+e],[0 1 1 1-e 1-e 0+e],c3);plot([0 1 1 0 0],[0 0 1 1 0]);disp('Weights');
  "IW{1,1}(48,:)'" : Constant  Value=[0.69868367682404952656582963754772208631038665771484375;0.186654436275727364513699058079509995877742767333984375;-0.5551675067174670630265609361231327056884765625;0.29542233086625302451722063779016025364398956298828125;0.413705506317406934702063381337211467325687408447265625;0.507571029405457618821628784644417464733123779296875;-0.91132337455524015101815393791184760630130767822265625;-0.281992313694674923141292310901917517185211181640625;0.452273541229704478805473399916081689298152923583984375;-1.0158316173242243340979484855779446661472320556640625]
      mask Display: e = 0.06;c1 = [120 150 230]/255;c2 = ([120 150 230]+0)/383;c3 = ([120 150 230]+128)/383;patch([0 1 1 0],[0 0 1 1],c1);patch([0 1 1 1-e 1-e 0+e],[0 0 1 1-e 0+e 0+e],c2);patch([0 0 1 1-e 0+e 0+e],[0 1 1 1-e 1-e 0+e],c3);plot([0 1 1 0 0],[0 0 1 1 0]);disp('Weights');
  "IW{1,1}(49,:)'" : Constant  Value=[-0.384007359998857544791661666749860160052776336669921875;-0.71047128787840529984265458551817573606967926025390625;0.710237209934762692142840023734606802463531494140625;-0.93633402362902395932309218551381491124629974365234375;0.62169053389579664870012720712111331522464752197265625;-0.75186685838180411511899592369445599615573883056640625;0.177732391685496204924987750928266905248165130615234375;0.1065736877580092667461286737307091243565082550048828125;0.9167768089996517488771132775582373142242431640625;0.841931106360764847096334051457233726978302001953125]
      mask Display: e = 0.06;c1 = [120 150 230]/255;c2 = ([120 150 230]+0)/383;c3 = ([120 150 230]+128)/383;patch([0 1 1 0],[0 0 1 1],c1);patch([0 1 1 1-e 1-e 0+e],[0 0 1 1-e 0+e 0+e],c2);patch([0 0 1 1-e 0+e 0+e],[0 1 1 1-e 1-e 0+e],c3);plot([0 1 1 0 0],[0 0 1 1 0]);disp('Weights');
  "IW{1,1}(5,:)'" : Constant  Value=[-0.09224594672063546330065264555742032825946807861328125;-0.38378360533188493608491853592568077147006988525390625;0.223639240732848965098611415669438429176807403564453125;0.276602420404264248698922301628044806420803070068359375;0.99449927835907292461570250452496111392974853515625;0.93383877466768672181984811686561442911624908447265625;-0.77997967173394344708725611781119368970394134521484375;0.94980856285733350485855908118537627160549163818359375;0.94553463289151185033887259123730473220348358154296875;-0.0222207631207075595458633188172825612127780914306640625]
      mask Display: e = 0.06;c1 = [120 150 230]/255;c2 = ([120 150 230]+0)/383;c3 = ([120 150 230]+128)/383;patch([0 1 1 0],[0 0 1 1],c1);patch([0 1 1 1-e 1-e 0+e],[0 0 1 1-e 0+e 0+e],c2);patch([0 0 1 1-e 0+e 0+e],[0 1 1 1-e 1-e 0+e],c3);plot([0 1 1 0 0],[0 0 1 1 0]);disp('Weights');
  "IW{1,1}(50,:)'" : Constant  Value=[-0.1679750521464102586133293470993521623313426971435546875;-0.865077149963036529101145788445137441158294677734375;0.67389365879715235063684986016596667468547821044921875;-0.6470971894533705803809198187082074582576751708984375;-0.5836682750283272991254079897771589457988739013671875;0.420528835051041216530620658886618912220001220703125;-0.8720034350370198250601561085204593837261199951171875;0.689747768182906728640091387205757200717926025390625;0.1388870772608765402633679286736878566443920135498046875;-0.81080414819806867487983481623814441263675689697265625]
      mask Display: e = 0.06;c1 = [120 150 230]/255;c2 = ([120 150 230]+0)/383;c3 = ([120 150 230]+128)/383;patch([0 1 1 0],[0 0 1 1],c1);patch([0 1 1 1-e 1-e 0+e],[0 0 1 1-e 0+e 0+e],c2);patch([0 0 1 1-e 0+e 0+e],[0 1 1 1-e 1-e 0+e],c3);plot([0 1 1 0 0],[0 0 1 1 0]);disp('Weights');
  "IW{1,1}(51,:)'" : Constant  Value=[0.44732261364571035411330512943095527589321136474609375;0.1758470803218625533315133679934660904109477996826171875;-0.233367352704531738627480308423400856554508209228515625;0.349371613537245995217972449609078466892242431640625;-0.90367897199846314304494399038958363234996795654296875;-0.478498032148415963771270753568387590348720550537109375;-0.64969492800252914843639473474468104541301727294921875;1.2003023143006663620013796389685012400150299072265625;1.1241909979501250038680382203892804682254791259765625;-0.6144687492976912412956380649120546877384185791015625]
      mask Display: e = 0.06;c1 = [120 150 230]/255;c2 = ([120 150 230]+0)/383;c3 = ([120 150 230]+128)/383;patch([0 1 1 0],[0 0 1 1],c1);patch([0 1 1 1-e 1-e 0+e],[0 0 1 1-e 0+e 0+e],c2);patch([0 0 1 1-e 0+e 0+e],[0 1 1 1-e 1-e 0+e],c3);plot([0 1 1 0 0],[0 0 1 1 0]);disp('Weights');
  "IW{1,1}(52,:)'" : Constant  Value=[-0.78819682681515190747489896239130757749080657958984375;0.388407732942888939131620418265811167657375335693359375;0.35989973075219394704760134118259884417057037353515625;0.66243263412910746712469745034468360245227813720703125;-0.015223181998556357952256945509361685253679752349853515625;-0.55855499675429876038634802171145565807819366455078125;-0.5733713000237565804440009742393158376216888427734375;0.91167693615170197762864745527622289955615997314453125;-0.7357307307862976930579179679625667631626129150390625;-0.90844078709634146218121486526797525584697723388671875]
      mask Display: e = 0.06;c1 = [120 150 230]/255;c2 = ([120 150 230]+0)/383;c3 = ([120 150 230]+128)/383;patch([0 1 1 0],[0 0 1 1],c1);patch([0 1 1 1-e 1-e 0+e],[0 0 1 1-e 0+e 0+e],c2);patch([0 0 1 1-e 0+e 0+e],[0 1 1 1-e 1-e 0+e],c3);plot([0 1 1 0 0],[0 0 1 1 0]);disp('Weights');
  "IW{1,1}(53,:)'" : Constant  Value=[0.71081224858643443642591819298104383051395416259765625;-0.69067337054457633715998099432908929884433746337890625;0.258485018155751256063723531042342074215412139892578125;0.7073769827294917877935631622676737606525421142578125;0.1627053995707752609423124567911145277321338653564453125;-0.264998526388344923798712216012063436210155487060546875;1.055188745046411469274971750564873218536376953125;-0.47513020219700641266769025605753995478153228759765625;-0.84711163547119927574868825104204006493091583251953125;-0.81798377747064054954506673311698250472545623779296875]
      mask Display: e = 0.06;c1 = [120 150 230]/255;c2 = ([120 150 230]+0)/383;c3 = ([120 150 230]+128)/383;patch([0 1 1 0],[0 0 1 1],c1);patch([0 1 1 1-e 1-e 0+e],[0 0 1 1-e 0+e 0+e],c2);patch([0 0 1 1-e 0+e 0+e],[0 1 1 1-e 1-e 0+e],c3);plot([0 1 1 0 0],[0 0 1 1 0]);disp('Weights');
  "IW{1,1}(54,:)'" : Constant  Value=[-0.8844130665775005173401268621091730892658233642578125;0.36312469072718922546982867061160504817962646484375;0.75033849106744099355381649729679338634014129638671875;0.09625505924436449090020317953531048260629177093505859375;0.72668641538420686298849204831640236079692840576171875;1.0379795885681117884047353072674013674259185791015625;-0.50402024763513775251766446672263555228710174560546875;0.407381459158563330458235896003316156566143035888671875;0.396630659984082589719633915592567063868045806884765625;-0.64648000798737925709502860627253539860248565673828125]
      mask Display: e = 0.06;c1 = [120 150 230]/255;c2 = ([120 150 230]+0)/383;c3 = ([120 150 230]+128)/383;patch([0 1 1 0],[0 0 1 1],c1);patch([0 1 1 1-e 1-e 0+e],[0 0 1 1-e 0+e 0+e],c2);patch([0 0 1 1-e 0+e 0+e],[0 1 1 1-e 1-e 0+e],c3);plot([0 1 1 0 0],[0 0 1 1 0]);disp('Weights');
  "IW{1,1}(55,:)'" : Constant  Value=[0.8176434584012703954414291729335673153400421142578125;-0.10935843617257516580121290417082491330802440643310546875;-1.0678496021682188921175793439033441245555877685546875;0.8030475963791838811545176213257946074008941650390625;-0.255839013256880409841187429265119135379791259765625;-1.2786444587533540850898816643166355788707733154296875;-0.183883969521893619880614778594463132321834564208984375;-0.0910435603925301706329520357030560262501239776611328125;0.22381954187360786345806218378129415214061737060546875;-0.46179159660903812412158231381908990442752838134765625]
      mask Display: e = 0.06;c1 = [120 150 230]/255;c2 = ([120 150 230]+0)/383;c3 = ([120 150 230]+128)/383;patch([0 1 1 0],[0 0 1 1],c1);patch([0 1 1 1-e 1-e 0+e],[0 0 1 1-e 0+e 0+e],c2);patch([0 0 1 1-e 0+e 0+e],[0 1 1 1-e 1-e 0+e],c3);plot([0 1 1 0 0],[0 0 1 1 0]);disp('Weights');
  "IW{1,1}(56,:)'" : Constant  Value=[0.1952193141698427003571936211301363073289394378662109375;0.402225719391471392416548269466147758066654205322265625;0.1036611251834579083830334411686635576188564300537109375;-0.1468207782462005173140795477593201212584972381591796875;-0.31994243490119866901721934482338838279247283935546875;-1.0496896435332054853262206961517222225666046142578125;-0.90612027769049541259249735958292149007320404052734375;-0.09067887520821189817343821459871833212673664093017578125;-0.99693300236474868825098383240401744842529296875;-0.26355133063217739408656825617072172462940216064453125]
      mask Display: e = 0.06;c1 = [120 150 230]/255;c2 = ([120 150 230]+0)/383;c3 = ([120 150 230]+128)/383;patch([0 1 1 0],[0 0 1 1],c1);patch([0 1 1 1-e 1-e 0+e],[0 0 1 1-e 0+e 0+e],c2);patch([0 0 1 1-e 0+e 0+e],[0 1 1 1-e 1-e 0+e],c3);plot([0 1 1 0 0],[0 0 1 1 0]);disp('Weights');
  "IW{1,1}(57,:)'" : Constant  Value=[-0.9493727955993092049169490564963780343532562255859375;-0.335615815333427158773105247746570967137813568115234375;0.2368186182419703411650147018008283339440822601318359375;0.7252467914222713307736967180971987545490264892578125;-0.428905396388163218102107521190191619098186492919921875;0.7210413471556280651242332169204019010066986083984375;0.11247903770765843578516296474845148622989654541015625;0.766090766262471856151705651427619159221649169921875;0.69547292458483467303409497617394663393497467041015625;1.0979280820838310805953597082407213747501373291015625]
      mask Display: e = 0.06;c1 = [120 150 230]/255;c2 = ([120 150 230]+0)/383;c3 = ([120 150 230]+128)/383;patch([0 1 1 0],[0 0 1 1],c1);patch([0 1 1 1-e 1-e 0+e],[0 0 1 1-e 0+e 0+e],c2);patch([0 0 1 1-e 0+e 0+e],[0 1 1 1-e 1-e 0+e],c3);plot([0 1 1 0 0],[0 0 1 1 0]);disp('Weights');
  "IW{1,1}(58,:)'" : Constant  Value=[0.94270674126308040552402189860004000365734100341796875;-0.135860400719931051494171470039873383939266204833984375;-1.05692479304946829188338597305119037628173828125;0.93612502985123169363390616126707755029201507568359375;0.0670282852011160057426053526796749792993068695068359375;0.68125601756195663938342477194964885711669921875;0.042234328149349742442808519626851193606853485107421875;0.388970644861843128925471546608605422079563140869140625;0.495188609801735901694286212659790180623531341552734375;-0.7962738885645552766590071769314818084239959716796875]
      mask Display: e = 0.06;c1 = [120 150 230]/255;c2 = ([120 150 230]+0)/383;c3 = ([120 150 230]+128)/383;patch([0 1 1 0],[0 0 1 1],c1);patch([0 1 1 1-e 1-e 0+e],[0 0 1 1-e 0+e 0+e],c2);patch([0 0 1 1-e 0+e 0+e],[0 1 1 1-e 1-e 0+e],c3);plot([0 1 1 0 0],[0 0 1 1 0]);disp('Weights');
  "IW{1,1}(59,:)'" : Constant  Value=[-0.8669523545897386274106111159198917448520660400390625;0.901720221085302142682849080301821231842041015625;-0.406824442344712100538828281059977598488330841064453125;-0.386446498945273109182352300194907002151012420654296875;-0.1953606819501915448089590654490166343748569488525390625;1.024995155631098331383554977946914732456207275390625;0.478714144885362957726471222485997714102268218994140625;-0.353616908023752396506012019017362035810947418212890625;1.0946616844466146023506780693423934280872344970703125;0.61289955389144623598696171029587276279926300048828125]
      mask Display: e = 0.06;c1 = [120 150 230]/255;c2 = ([120 150 230]+0)/383;c3 = ([120 150 230]+128)/383;patch([0 1 1 0],[0 0 1 1],c1);patch([0 1 1 1-e 1-e 0+e],[0 0 1 1-e 0+e 0+e],c2);patch([0 0 1 1-e 0+e 0+e],[0 1 1 1-e 1-e 0+e],c3);plot([0 1 1 0 0],[0 0 1 1 0]);disp('Weights');
  "IW{1,1}(6,:)'" : Constant  Value=[-1.1437587265543982528726019154419191181659698486328125;-1.1455093095544304215849251704639755189418792724609375;-0.42315702137301214325049159015179611742496490478515625;-0.79131674418211961352653815993107855319976806640625;0.50078581960100765346766138463863171637058258056640625;0.64058661303697073119423066600575111806392669677734375;-0.401792931913857731540673512427019886672496795654296875;0.35925804829260632455856239175773225724697113037109375;-0.5222730813321685428007867812993936240673065185546875;0.966781856970008401930272157187573611736297607421875]
      mask Display: e = 0.06;c1 = [120 150 230]/255;c2 = ([120 150 230]+0)/383;c3 = ([120 150 230]+128)/383;patch([0 1 1 0],[0 0 1 1],c1);patch([0 1 1 1-e 1-e 0+e],[0 0 1 1-e 0+e 0+e],c2);patch([0 0 1 1-e 0+e 0+e],[0 1 1 1-e 1-e 0+e],c3);plot([0 1 1 0 0],[0 0 1 1 0]);disp('Weights');
  "IW{1,1}(60,:)'" : Constant  Value=[0.3590401829143894385509838684811256825923919677734375;-0.203844352651413707189220758664305321872234344482421875;-0.028674353306721182821359406034389394335448741912841796875;0.1898780270719273299828699919089558534324169158935546875;-0.97107737206335542623492074199020862579345703125;-0.7049470997716416054146293390658684074878692626953125;0.041026748217958097786350890601170249283313751220703125;-1.0857285954157307461542814053245820105075836181640625;-0.413997771209523357516246733212028630077838897705078125;-0.94522664251705579285811609224765561521053314208984375]
      mask Display: e = 0.06;c1 = [120 150 230]/255;c2 = ([120 150 230]+0)/383;c3 = ([120 150 230]+128)/383;patch([0 1 1 0],[0 0 1 1],c1);patch([0 1 1 1-e 1-e 0+e],[0 0 1 1-e 0+e 0+e],c2);patch([0 0 1 1-e 0+e 0+e],[0 1 1 1-e 1-e 0+e],c3);plot([0 1 1 0 0],[0 0 1 1 0]);disp('Weights');
  "IW{1,1}(61,:)'" : Constant  Value=[-0.64035559688825760549235610596952028572559356689453125;0.74513611107510546727183964321739040315151214599609375;-0.7848448124750111443148625767207704484462738037109375;0.73062370659019337804096494437544606626033782958984375;-1.327406872915831481662962687551043927669525146484375;0.44985153691166879230678432577406056225299835205078125;0.242066233793844898247726860063266940414905548095703125;-0.13318329333336986763924869592301547527313232421875;-1.0857085629759186673481963225640356540679931640625;-0.43370504020426292601797513270867057144641876220703125]
      mask Display: e = 0.06;c1 = [120 150 230]/255;c2 = ([120 150 230]+0)/383;c3 = ([120 150 230]+128)/383;patch([0 1 1 0],[0 0 1 1],c1);patch([0 1 1 1-e 1-e 0+e],[0 0 1 1-e 0+e 0+e],c2);patch([0 0 1 1-e 0+e 0+e],[0 1 1 1-e 1-e 0+e],c3);plot([0 1 1 0 0],[0 0 1 1 0]);disp('Weights');
  "IW{1,1}(62,:)'" : Constant  Value=[0.56247112982970903782842242435435764491558074951171875;-0.74969872442936613676778279113932512700557708740234375;-0.29933358265625631400297379514086060225963592529296875;0.558077793128705312852844144799746572971343994140625;-1.0314085660909235730997579594259150326251983642578125;-0.96914425047493291121014635791652835905551910400390625;-0.78641950874881827449058846468687988817691802978515625;0.70710463178118965199558942913427017629146575927734375;-0.7120509947509050530101148979156278073787689208984375;0.0661142240607381082018179085935116745531558990478515625]
      mask Display: e = 0.06;c1 = [120 150 230]/255;c2 = ([120 150 230]+0)/383;c3 = ([120 150 230]+128)/383;patch([0 1 1 0],[0 0 1 1],c1);patch([0 1 1 1-e 1-e 0+e],[0 0 1 1-e 0+e 0+e],c2);patch([0 0 1 1-e 0+e 0+e],[0 1 1 1-e 1-e 0+e],c3);plot([0 1 1 0 0],[0 0 1 1 0]);disp('Weights');
  "IW{1,1}(63,:)'" : Constant  Value=[0.2036535758647045335489877970758243463933467864990234375;0.18824162646012132515949133448884822428226470947265625;0.055030042589781870410181596753318444825708866119384765625;-0.1219277958454305366142733646483975462615489959716796875;0.93690798210580006344372350213234312832355499267578125;0.57814017757580604683909086816129274666309356689453125;0.9188476004671548569291417152271606028079986572265625;0.54028752991031703256652463096543215215206146240234375;0.1502869953193684826597831261096871457993984222412109375;0.8562197272430813743682165295467711985111236572265625]
      mask Display: e = 0.06;c1 = [120 150 230]/255;c2 = ([120 150 230]+0)/383;c3 = ([120 150 230]+128)/383;patch([0 1 1 0],[0 0 1 1],c1);patch([0 1 1 1-e 1-e 0+e],[0 0 1 1-e 0+e 0+e],c2);patch([0 0 1 1-e 0+e 0+e],[0 1 1 1-e 1-e 0+e],c3);plot([0 1 1 0 0],[0 0 1 1 0]);disp('Weights');
  "IW{1,1}(64,:)'" : Constant  Value=[-0.9100771309814212894906404471839778125286102294921875;-0.666302301310716327265026848181150853633880615234375;-0.460355056312492738612718312651850283145904541015625;0.52572845760131858838803964317776262760162353515625;0.92898705103636747271167450890061445534229278564453125;-0.456615502282086083152279343266854993999004364013671875;0.72570389526679590641577988208155147731304168701171875;0.8739902853463608067841050797142088413238525390625;0.1586716700514758382478675002857926301658153533935546875;-0.08265304627885201871340115076236543245613574981689453125]
      mask Display: e = 0.06;c1 = [120 150 230]/255;c2 = ([120 150 230]+0)/383;c3 = ([120 150 230]+128)/383;patch([0 1 1 0],[0 0 1 1],c1);patch([0 1 1 1-e 1-e 0+e],[0 0 1 1-e 0+e 0+e],c2);patch([0 0 1 1-e 0+e 0+e],[0 1 1 1-e 1-e 0+e],c3);plot([0 1 1 0 0],[0 0 1 1 0]);disp('Weights');
  "IW{1,1}(7,:)'" : Constant  Value=[-0.6011493278455954936134730814956128597259521484375;-0.94397276205370861390520076383836567401885986328125;-0.63936467363710303146717706113122403621673583984375;-0.323930740023200269828151931505999527871608734130859375;0.8082167859878934823569807122112251818180084228515625;-0.995454398462420453341792381252162158489227294921875;0.84903160133359578676248702322482131421566009521484375;-0.1782502368205074183560299161399598233401775360107421875;0.1794540570386025934990215091602294705808162689208984375;0.356538739670403559411937521872459910809993743896484375]
      mask Display: e = 0.06;c1 = [120 150 230]/255;c2 = ([120 150 230]+0)/383;c3 = ([120 150 230]+128)/383;patch([0 1 1 0],[0 0 1 1],c1);patch([0 1 1 1-e 1-e 0+e],[0 0 1 1-e 0+e 0+e],c2);patch([0 0 1 1-e 0+e 0+e],[0 1 1 1-e 1-e 0+e],c3);plot([0 1 1 0 0],[0 0 1 1 0]);disp('Weights');
  "IW{1,1}(8,:)'" : Constant  Value=[-0.83428521927244070344187321097706444561481475830078125;0.35537394497407337468075638753361999988555908203125;0.6093596734300064099443261511623859405517578125;-1.132505948065638090582751829060725867748260498046875;0.536982872837481917116519980481825768947601318359375;-0.7799684295941042844191315452917478978633880615234375;0.33586439695868453014782062382437288761138916015625;-0.97318600109317543456199928186833858489990234375;-0.172659258810985871690490967012010514736175537109375;0.4270377686523072480184737287345342338085174560546875]
      mask Display: e = 0.06;c1 = [120 150 230]/255;c2 = ([120 150 230]+0)/383;c3 = ([120 150 230]+128)/383;patch([0 1 1 0],[0 0 1 1],c1);patch([0 1 1 1-e 1-e 0+e],[0 0 1 1-e 0+e 0+e],c2);patch([0 0 1 1-e 0+e 0+e],[0 1 1 1-e 1-e 0+e],c3);plot([0 1 1 0 0],[0 0 1 1 0]);disp('Weights');
  "IW{1,1}(9,:)'" : Constant  Value=[-0.49154311227124203309557515240157954394817352294921875;0.70347695075763005956304141363943926990032196044921875;-0.051520579344400518895241702921339310705661773681640625;0.6370740768855644997614717794931493699550628662109375;0.56851958404243474465289409636170603334903717041015625;-1.0275247477109650251492212191806174814701080322265625;-0.49961662332965872668211204654653556644916534423828125;-0.83957038265836791968155239374027587473392486572265625;0.6781097209942430481532937847077846527099609375;-0.9678398189212373825540680627455003559589385986328125]
      mask Display: e = 0.06;c1 = [120 150 230]/255;c2 = ([120 150 230]+0)/383;c3 = ([120 150 230]+128)/383;patch([0 1 1 0],[0 0 1 1],c1);patch([0 1 1 1-e 1-e 0+e],[0 0 1 1-e 0+e 0+e],c2);patch([0 0 1 1-e 0+e 0+e],[0 1 1 1-e 1-e 0+e],c3);plot([0 1 1 0 0],[0 0 1 1 0]);disp('Weights');
  Mux : Mux  Inputs=64
      mask Display: e = 0.06;c1 = [120 150 230]/255;c2 = ([120 150 230]+0)/383;c3 = ([120 150 230]+128)/383;patch([0 1 1 0],[0 0 1 1],c1);patch([0 1 1 1-e 1-e 0+e],[0 0 1 1-e 0+e 0+e],c2);patch([0 0 1 1-e 0+e 0+e],[0 1 1 1-e 1-e 0+e],c3);plot([0 1 1 0 0],[0 0 1 1 0]);disp('Mux');
  dotprod{1..64} (64 alike) : neural/Weight Functions/dotprod
  "iz{1,1}" : Outport
      mask Display: e = 0.06;c1 = [120 230 180]/255;c2 = ([120 230 180]+0)/(256+128);c3 = ([120 230 180]+128)/(256+128);patch([0 1 1 0],[0 0 1 1],c1);patch([0 1 1 1-e 1-e 0+e],[0 0 1 1-e 0+e 0+e],c2);patch([0 0 1 1-e 0+e 0+e],[0 1 1 1-e 1-e 0+e],c3);plot([0 1 1 0 0],[0 0 1 1 0]);
  wires:
  "IW{1,1}(1,:)'"/1 -> dotprod1/1
  "pd{1,1}"/1 -> dotprod1/2, dotprod2/2, dotprod3/2, dotprod4/2, dotprod5/2, dotprod6/2, dotprod7/2, dotprod8/2, dotprod9/2, dotprod10/2, dotprod11/2, dotprod12/2, dotprod13/2, dotprod14/2, dotprod15/2, dotprod16/2, dotprod17/2, dotprod18/2, dotprod19/2, dotprod20/2, dotprod21/2, dotprod22/2, dotprod23/2, dotprod24/2, dotprod25/2, dotprod26/2, dotprod27/2, dotprod28/2, dotprod29/2, dotprod30/2, dotprod31/2, dotprod32/2, dotprod33/2, dotprod34/2, dotprod35/2, dotprod36/2, dotprod37/2, dotprod38/2, dotprod39/2, dotprod40/2, dotprod41/2, dotprod42/2, dotprod43/2, dotprod44/2, dotprod45/2, dotprod46/2, dotprod47/2, dotprod48/2, dotprod49/2, dotprod50/2, dotprod51/2, dotprod52/2, dotprod53/2, dotprod54/2, dotprod55/2, dotprod56/2, dotprod57/2, dotprod58/2, dotprod59/2, dotprod60/2, dotprod61/2, dotprod62/2, dotprod63/2, dotprod64/2
  dotprod1/1 -> Mux/1
  "IW{1,1}(2,:)'"/1 -> dotprod2/1
  dotprod2/1 -> Mux/2
  "IW{1,1}(3,:)'"/1 -> dotprod3/1
  dotprod3/1 -> Mux/3
  "IW{1,1}(4,:)'"/1 -> dotprod4/1
  dotprod4/1 -> Mux/4
  "IW{1,1}(5,:)'"/1 -> dotprod5/1
  dotprod5/1 -> Mux/5
  "IW{1,1}(6,:)'"/1 -> dotprod6/1
  dotprod6/1 -> Mux/6
  "IW{1,1}(7,:)'"/1 -> dotprod7/1
  dotprod7/1 -> Mux/7
  "IW{1,1}(8,:)'"/1 -> dotprod8/1
  dotprod8/1 -> Mux/8
  "IW{1,1}(9,:)'"/1 -> dotprod9/1
  dotprod9/1 -> Mux/9
  "IW{1,1}(10,:)'"/1 -> dotprod10/1
  dotprod10/1 -> Mux/10
  "IW{1,1}(11,:)'"/1 -> dotprod11/1
  dotprod11/1 -> Mux/11
  "IW{1,1}(12,:)'"/1 -> dotprod12/1
  dotprod12/1 -> Mux/12
  "IW{1,1}(13,:)'"/1 -> dotprod13/1
  dotprod13/1 -> Mux/13
  "IW{1,1}(14,:)'"/1 -> dotprod14/1
  dotprod14/1 -> Mux/14
  "IW{1,1}(15,:)'"/1 -> dotprod15/1
  dotprod15/1 -> Mux/15
  "IW{1,1}(16,:)'"/1 -> dotprod16/1
  dotprod16/1 -> Mux/16
  "IW{1,1}(17,:)'"/1 -> dotprod17/1
  dotprod17/1 -> Mux/17
  "IW{1,1}(18,:)'"/1 -> dotprod18/1
  dotprod18/1 -> Mux/18
  "IW{1,1}(19,:)'"/1 -> dotprod19/1
  dotprod19/1 -> Mux/19
  "IW{1,1}(20,:)'"/1 -> dotprod20/1
  dotprod20/1 -> Mux/20
  "IW{1,1}(21,:)'"/1 -> dotprod21/1
  dotprod21/1 -> Mux/21
  "IW{1,1}(22,:)'"/1 -> dotprod22/1
  dotprod22/1 -> Mux/22
  "IW{1,1}(23,:)'"/1 -> dotprod23/1
  dotprod23/1 -> Mux/23
  "IW{1,1}(24,:)'"/1 -> dotprod24/1
  dotprod24/1 -> Mux/24
  "IW{1,1}(25,:)'"/1 -> dotprod25/1
  dotprod25/1 -> Mux/25
  "IW{1,1}(26,:)'"/1 -> dotprod26/1
  dotprod26/1 -> Mux/26
  "IW{1,1}(27,:)'"/1 -> dotprod27/1
  dotprod27/1 -> Mux/27
  "IW{1,1}(28,:)'"/1 -> dotprod28/1
  dotprod28/1 -> Mux/28
  "IW{1,1}(29,:)'"/1 -> dotprod29/1
  dotprod29/1 -> Mux/29
  "IW{1,1}(30,:)'"/1 -> dotprod30/1
  dotprod30/1 -> Mux/30
  "IW{1,1}(31,:)'"/1 -> dotprod31/1
  dotprod31/1 -> Mux/31
  "IW{1,1}(32,:)'"/1 -> dotprod32/1
  dotprod32/1 -> Mux/32
  "IW{1,1}(33,:)'"/1 -> dotprod33/1
  dotprod33/1 -> Mux/33
  "IW{1,1}(34,:)'"/1 -> dotprod34/1
  dotprod34/1 -> Mux/34
  "IW{1,1}(35,:)'"/1 -> dotprod35/1
  dotprod35/1 -> Mux/35
  "IW{1,1}(36,:)'"/1 -> dotprod36/1
  dotprod36/1 -> Mux/36
  "IW{1,1}(37,:)'"/1 -> dotprod37/1
  dotprod37/1 -> Mux/37
  "IW{1,1}(38,:)'"/1 -> dotprod38/1
  dotprod38/1 -> Mux/38
  "IW{1,1}(39,:)'"/1 -> dotprod39/1
  dotprod39/1 -> Mux/39
  "IW{1,1}(40,:)'"/1 -> dotprod40/1
  dotprod40/1 -> Mux/40
  "IW{1,1}(41,:)'"/1 -> dotprod41/1
  dotprod41/1 -> Mux/41
  "IW{1,1}(42,:)'"/1 -> dotprod42/1
  dotprod42/1 -> Mux/42
  "IW{1,1}(43,:)'"/1 -> dotprod43/1
  dotprod43/1 -> Mux/43
  "IW{1,1}(44,:)'"/1 -> dotprod44/1
  dotprod44/1 -> Mux/44
  "IW{1,1}(45,:)'"/1 -> dotprod45/1
  dotprod45/1 -> Mux/45
  "IW{1,1}(46,:)'"/1 -> dotprod46/1
  dotprod46/1 -> Mux/46
  "IW{1,1}(47,:)'"/1 -> dotprod47/1
  dotprod47/1 -> Mux/47
  "IW{1,1}(48,:)'"/1 -> dotprod48/1
  dotprod48/1 -> Mux/48
  "IW{1,1}(49,:)'"/1 -> dotprod49/1
  dotprod49/1 -> Mux/49
  "IW{1,1}(50,:)'"/1 -> dotprod50/1
  dotprod50/1 -> Mux/50
  "IW{1,1}(51,:)'"/1 -> dotprod51/1
  dotprod51/1 -> Mux/51
  "IW{1,1}(52,:)'"/1 -> dotprod52/1
  dotprod52/1 -> Mux/52
  "IW{1,1}(53,:)'"/1 -> dotprod53/1
  dotprod53/1 -> Mux/53
  "IW{1,1}(54,:)'"/1 -> dotprod54/1
  dotprod54/1 -> Mux/54
  "IW{1,1}(55,:)'"/1 -> dotprod55/1
  dotprod55/1 -> Mux/55
  "IW{1,1}(56,:)'"/1 -> dotprod56/1
  dotprod56/1 -> Mux/56
  "IW{1,1}(57,:)'"/1 -> dotprod57/1
  dotprod57/1 -> Mux/57
  "IW{1,1}(58,:)'"/1 -> dotprod58/1
  dotprod58/1 -> Mux/58
  "IW{1,1}(59,:)'"/1 -> dotprod59/1
  dotprod59/1 -> Mux/59
  "IW{1,1}(60,:)'"/1 -> dotprod60/1
  dotprod60/1 -> Mux/60
  "IW{1,1}(61,:)'"/1 -> dotprod61/1
  dotprod61/1 -> Mux/61
  "IW{1,1}(62,:)'"/1 -> dotprod62/1
  dotprod62/1 -> Mux/62
  "IW{1,1}(63,:)'"/1 -> dotprod63/1
  dotprod63/1 -> Mux/63
  "IW{1,1}(64,:)'"/1 -> dotprod64/1
  dotprod64/1 -> Mux/64
  Mux/1 -> "iz{1,1}"/1
